simulink model "DSPequivalent_IM"  (R2018b)
settings: Solver=ode5  StartTime=0.0  StopTime=0.15  FixedStep=Tsim  RelTol=1e-3
values from neighbouring files (symbols this model uses):
  DEADTIME = 100    [init_DSPeq_FOC.m]    (also in init_DSPeq_IM.m)
  f_ref = 270    [init_DSPeq_FOC.m]    (also in init_DSPeq_IM.m = 50)
  Id_ref = 0    [init_DSPeq_FOC.m]    (also in init_DSPeq_IM.m = 1; step_prikaz.m = Idq2(:,2))
  Iq_ref = 2    [init_DSPeq_FOC.m]    (also in init_DSPeq_IM.m = 1; step_prikaz.m = Idq2(:,3))
  ISENSE_SCALE = 10    [init_DSPeq_FOC.m]    (also in init_DSPeq_IM.m)
  J = 15e-3    (= 0.015)    [init_DSPeq_IM.m]
  K1 = alpha*L/Ts    (= 68.108974359)    [init_DSPeq_FOC.m]    (also in init_DSPeq_IM.m = 301.121794872)
  K2 = exp(-Ts/taus)    [init_DSPeq_FOC.m]    (also in init_DSPeq_IM.m = exp(-Ts*Rs/Ls))
  Lge = (Ls*Lr-Lm^2)/Lr    (= 0.0459761697497)    [init_DSPeq_IM.m]
  Lm = 0.3482    [init_DSPeq_IM.m]
  Lr = Lm + Lgr    (= 0.3676)    [init_DSPeq_IM.m]
  Nos = 16    [init_DSPeq.m]    (also in init_DSPeq_FOC.m; init_DSPeq_IM.m)
  OVERSAMPLING = 1    [init_DSPeq.m]    (also in init_DSPeq_FOC.m; init_DSPeq_IM.m; raw_plot.m)
  p = 3    [init_DSPeq_FOC.m]    (also in init_DSPeq_IM.m = 1)
  PWM_TBPRD = 4992    [init_DSPeq.m]    (also in init_DSPeq_FOC.m; init_DSPeq_IM.m; paramSet.m)
  Rr = 11.202    [init_DSPeq_IM.m]
  Rs = 10    [init_DSPeq.m]    (also in init_DSPeq_IM.m = 13.12)
  Tadc = Tpwm/Nos    (= 6.24e-06)    [init_DSPeq.m]    (also in init_DSPeq_FOC.m; init_DSPeq_IM.m)
  Tpwm = 2*PWM_TBPRD/ftbclk    (= 9.984e-05)    [init_DSPeq.m]    (also in init_DSPeq_FOC.m; init_DSPeq_IM.m; paramSet.m)
  Ts = Tpwm/ur    (= 2.496e-05)    [init_DSPeq.m]    (also in init_DSPeq_FOC.m = 1.248e-05; init_DSPeq_IM.m = 4.992e-05; paramSet.m = 4.992e-05; step_prikaz.m = Ts/1000)
  Ttbclk = 1/ftbclk    (= 1e-08)    [init_DSPeq.m]    (also in init_DSPeq_FOC.m; init_DSPeq_IM.m; paramSet.m)
  UD_MAX = Udq_max    [init_DSPeq_IM.m]
  UD_MIN = -Udq_max    [init_DSPeq_IM.m]
  Udol = 0    [init_DSPeq_FOC.m]    (also in init_DSPeq_IM.m = UD_MAX/2)
  UQ_MAX = Udq_max    [init_DSPeq_IM.m]
  UQ_MIN = -Udq_max    [init_DSPeq_IM.m]
  Uqol = 0    [init_DSPeq_FOC.m]    (also in init_DSPeq_IM.m)
  ur = 4    [init_DSPeq.m]    (also in init_DSPeq_FOC.m = 8; init_DSPeq_IM.m = 2; paramSet.m = 2; raw_plot.m = 2)
libraries: simulink x7, simulink_extras x1
settings Model: Creator=ruzic  LastModifiedBy=ruzic
settings DebuggingCC: UnderSpecifiedDataTypeMsg=warning  UnderSpecifiedDimensionMsg=warning

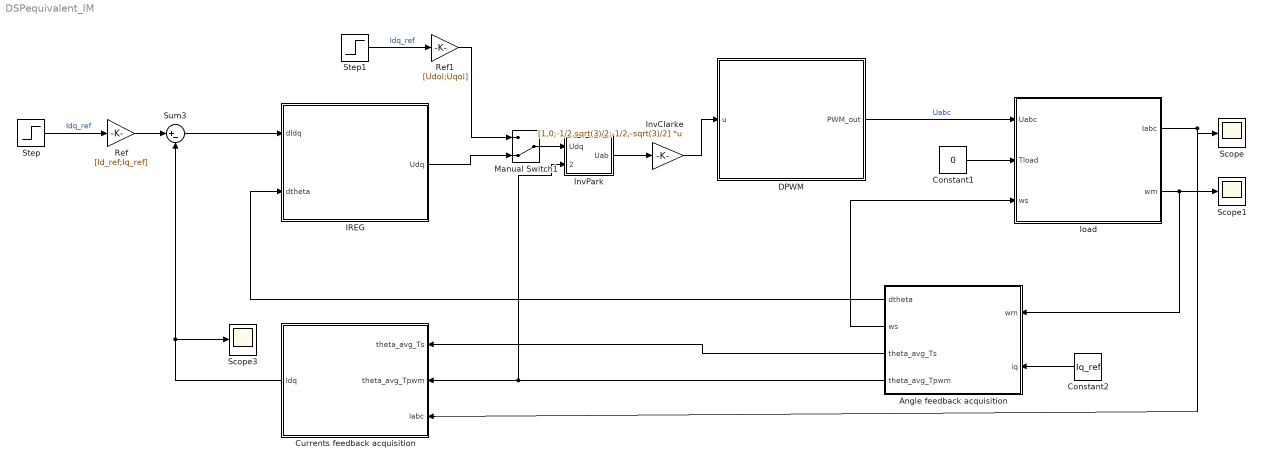
== system DSPequivalent_IM ==
  Angle feedback acquisition : Subsystem
  Constant1 : Constant  Value=0
  Constant2 : Constant  Value=Iq_ref
  Currents feedback acquisition : Subsystem
  DPWM : Subsystem
  IREG : Subsystem
  InvClarke : Gain  Gain=[1,0;-1/2,sqrt(3)/2;-1/2,-sqrt(3)/2]  Multiplication=Matrix(K*u)
  InvPark : Subsystem
  Manual Switch1 : ManualSwitch  CurrentSetting=0
  Ref : Gain  Gain=[Id_ref;Iq_ref]
  Ref1 : Gain  Gain=[Udol;Uqol]
  Scope : Scope
  Scope1 : Scope
  Scope3 : Scope
  Step : Step  Time=Tpwm/ur  SampleTime=Ts
  Step1 : Step  Time=Tpwm/ur  SampleTime=Ts
  Sum3 : Sum  Inputs=|+-
  load : Subsystem
  wires:
  Sum3/1 -> IREG/1(dIdq)
  Step/1 -> Ref/1  "Idq_ref"
  DPWM/1(PWM_out) -> load/1(Uabc)  "Uabc"
  load/1(Iabc) -> Scope/1, Currents feedback acquisition/3(Iabc)
  Ref1/1 -> Manual Switch1/1
  InvPark/1(Uab) -> InvClarke/1
  InvClarke/1 -> DPWM/1(u)
  Ref/1 -> Sum3/1
  Step1/1 -> Ref1/1  "Idq_ref"
  Currents feedback acquisition/1("Idq ") -> Scope3/1, Sum3/2
  IREG/1(Udq) -> Manual Switch1/2
  Manual Switch1/1 -> InvPark/1(Udq)
  Constant1/1 -> load/2(Tload)
  Angle feedback acquisition/4(theta_avg_Tpwm) -> Currents feedback acquisition/2(theta_avg_Tpwm), InvPark/2(theta)
  Angle feedback acquisition/1(dtheta) -> IREG/2(dtheta)
  Angle feedback acquisition/2(ws) -> load/3(ws)
  Angle feedback acquisition/3(theta_avg_Ts) -> Currents feedback acquisition/1(theta_avg_Ts)
  Constant2/1 -> Angle feedback acquisition/2(iq)
  load/2(wm) -> Angle feedback acquisition/1(wm), Scope1/1

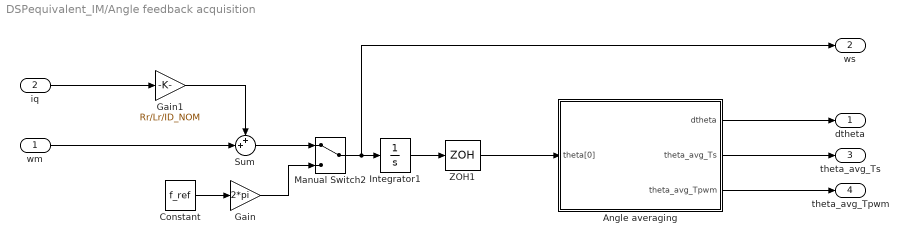
== system DSPequivalent_IM/Angle feedback acquisition ==
  wm : Inport
  iq : Inport  Port=2
  Angle averaging : Subsystem
  Constant : Constant  Value=f_ref
  Gain : Gain  Gain=2*pi
  Gain1 : Gain  Gain=Rr/Lr/ID_NOM
  Integrator1 : Integrator  WrapState=on  WrappedStateUpperValue=2*pi  WrappedStateLowerValue=0
  Manual Switch2 : ManualSwitch
  Sum : Sum  Inputs=++|
  ZOH1 : ZeroOrderHold  SampleTime=Ts
  dtheta : Outport
  ws : Outport  Port=2
  theta_avg_Ts : Outport  Port=3
  theta_avg_Tpwm : Outport  Port=4
  wires:
  ZOH1/1 -> Angle averaging/1(theta[0])
  Gain1/1 -> Sum/1
  iq/1 -> Gain1/1
  Sum/1 -> Manual Switch2/1
  Constant/1 -> Gain/1
  Manual Switch2/1 -> ws/1, Integrator1/1
  Gain/1 -> Manual Switch2/2
  Angle averaging/2(theta_avg_Ts) -> theta_avg_Ts/1
  Integrator1/1 -> ZOH1/1
  Angle averaging/3(theta_avg_Tpwm) -> theta_avg_Tpwm/1
  Angle averaging/1(dtheta) -> dtheta/1
  wm/1 -> Sum/2

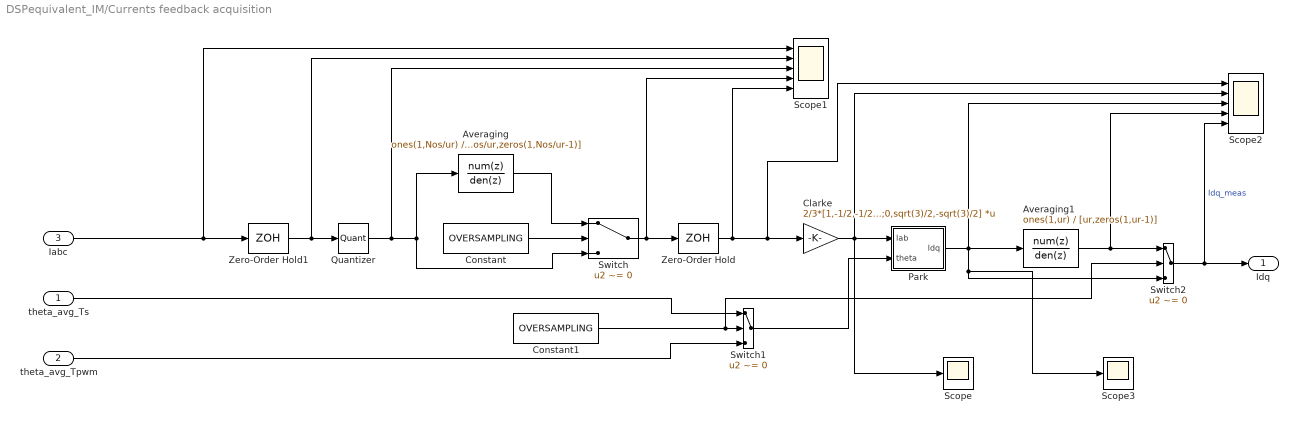
== system DSPequivalent_IM/Currents feedback acquisition ==
  theta_avg_Ts : Inport
  theta_avg_Tpwm : Inport  Port=2
  Iabc : Inport  Port=3
  Averaging : DiscreteTransferFcn  Numerator=ones(1,Nos/ur)  Denominator=[Nos/ur,zeros(1,Nos/ur-1)]
  Averaging1 : DiscreteTransferFcn  Numerator=ones(1,ur)  Denominator=[ur,zeros(1,ur-1)]
  Clarke : Gain  Gain=2/3*[1,-1/2,-1/2;0,sqrt(3)/2,-sqrt(3)/2]  Multiplication=Matrix(K*u)
  Constant : Constant  Value=OVERSAMPLING
  Constant1 : Constant  Value=OVERSAMPLING
  Park : Subsystem
  Quantizer : Quantizer  QuantizationInterval=3/(2^12-1)*ISENSE_SCALE
  Scope : Scope
  Scope1 : Scope  NumInputPorts=5
  Scope2 : Scope  NumInputPorts=5
  Scope3 : Scope
  Switch : Switch  Criteria=u2 ~= 0
  Switch1 : Switch  Criteria=u2 ~= 0
  Switch2 : Switch  Criteria=u2 ~= 0
  Zero-Order Hold : ZeroOrderHold  SampleTime=Ts
  Zero-Order Hold1 : ZeroOrderHold  SampleTime=Tadc
  "Idq " : Outport
  wires:
  Iabc/1 -> Zero-Order Hold1/1, Scope1/1
  Switch/1 -> Scope1/4, Zero-Order Hold/1
  Zero-Order Hold1/1 -> Quantizer/1, Scope1/2
  Quantizer/1 -> Switch/3, Averaging/1, Scope1/3
  Averaging/1 -> Switch/1
  Constant/1 -> Switch/2
  Constant1/1 -> Switch2/2, Switch1/2
  Switch2/1 -> Scope2/5, "Idq "/1  "Idq_meas"
  theta_avg_Tpwm/1 -> Switch1/3
  theta_avg_Ts/1 -> Switch1/1
  Averaging1/1 -> Scope2/4, Switch2/1
  Switch1/1 -> Park/2(theta)
  Clarke/1 -> Scope/1, Scope2/2, Park/1(Iab)
  Park/1(Idq) -> Scope2/3, Averaging1/1, Scope3/1, Switch2/3
  Zero-Order Hold/1 -> Scope2/1, Clarke/1, Scope1/5

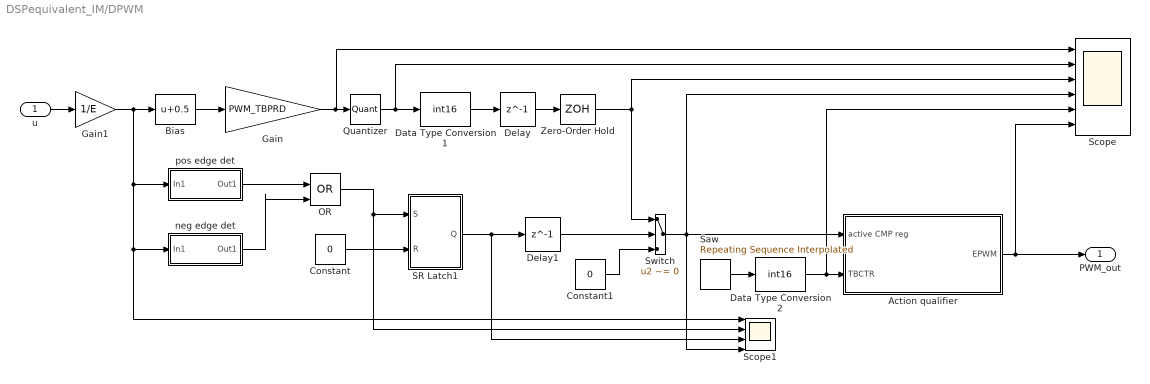
== system DSPequivalent_IM/DPWM ==
  u : Inport
  Action qualifier : Subsystem
  Bias : Bias  Bias=0.5
  Constant : Constant  Value=0
  Constant1 : Constant  Value=0
  Data Type Conversion1 : DataTypeConversion  OutDataTypeStr=int16  ConvertRealWorld=Stored Integer (SI)  RndMeth=Round
  Data Type Conversion2 : DataTypeConversion  OutDataTypeStr=int16  ConvertRealWorld=Stored Integer (SI)  RndMeth=Round
  Delay : Delay  DelayLength=1  SampleTime=Ts
  Delay1 : Delay  DelayLength=1  SampleTime=Ts
  Gain : Gain  Gain=PWM_TBPRD
  Gain1 : Gain  Gain=1/E
  OR : Logic  Operator=OR  IconShape=distinctive  AllPortsSameDT=off  OutDataTypeStr=boolean
  Quantizer : Quantizer  QuantizationInterval=1
  SR Latch1 : Subsystem
  Saw : simulink/Sources/Repeating Sequence Interpolated  OutValues=[0 PWM_TBPRD 1].'  TimeValues=[0 Tpwm/2 (Tpwm-Ttbclk)].'  LookUpMeth=Interpolation-Use End Values  tsamp=Ttbclk  OutMin=[]  OutMax=[]  OutDataTypeStr=double  OutputDataTypeScalingMode=double  OutDataType=fixdt(0,8)  OutScaling=2^-10
  Scope : Scope  NumInputPorts=6
  Scope1 : Scope  NumInputPorts=4
  Switch : Switch  Criteria=u2 ~= 0
  Zero-Order Hold : ZeroOrderHold  SampleTime=-1
  neg edge det : Subsystem
  pos edge det : Subsystem
  PWM_out : Outport
  wires:
  u/1 -> Gain1/1
  Quantizer/1 -> Data Type Conversion1/1, Scope/2
  Saw/1 -> Data Type Conversion2/1
  Switch/1 -> Scope/4, Action qualifier/1(active CMP reg), Scope1/4
  Action qualifier/1(EPWM) -> Scope/6, PWM_out/1
  Data Type Conversion1/1 -> Delay/1
  Data Type Conversion2/1 -> Scope/5, Action qualifier/2(TBCTR)
  Gain1/1 -> Scope1/1, neg edge det/1(In1), pos edge det/1(In1), Bias/1
  Gain/1 -> Scope/1, Quantizer/1
  Constant/1 -> SR Latch1/2(R)
  neg edge det/1(Out1) -> OR/2
  pos edge det/1(Out1) -> OR/1
  OR/1 -> Scope1/2, SR Latch1/1(S)
  SR Latch1/1(Q) -> Scope1/3, Delay1/1
  Constant1/1 -> Switch/3
  Bias/1 -> Gain/1
  Delay/1 -> Zero-Order Hold/1
  Zero-Order Hold/1 -> Scope/3, Switch/1
  Delay1/1 -> Switch/2

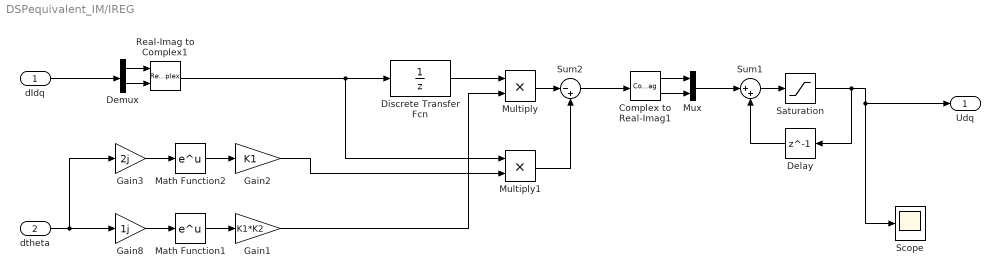
== system DSPequivalent_IM/IREG ==
  dIdq : Inport
  dtheta : Inport  Port=2
  Complex to Real-Imag1 : ComplexToRealImag
  Delay : Delay  DelayLength=1
  Demux : Demux  Outputs=2
  Discrete Transfer Fcn : DiscreteTransferFcn  Denominator=[1 0]
  Gain1 : Gain  Gain=K1*K2
  Gain2 : Gain  Gain=K1
  Gain3 : Gain  Gain=2j
  Gain8 : Gain  Gain=1j
  Math Function1 : Math  OutputSignalType=complex  SaturateOnIntegerOverflow=on
  Math Function2 : Math  OutputSignalType=complex  SaturateOnIntegerOverflow=on
  Multiply : Product
  Multiply1 : Product
  Mux : Mux  Inputs=2
  Real-Imag to Complex1 : RealImagToComplex
  Saturation : Saturate  UpperLimit=[UD_MAX; UQ_MAX]  LowerLimit=[UD_MIN; UQ_MIN]
  Scope : Scope
  Sum1 : Sum  Inputs=|++
  Sum2 : Sum  Inputs=|-+
  Udq : Outport
  wires:
  Saturation/1 -> Udq/1, Scope/1, Delay/1
  Sum1/1 -> Saturation/1
  Delay/1 -> Sum1/2
  Demux/2 -> Real-Imag to Complex1/2
  Math Function1/1 -> Gain1/1
  Mux/1 -> Sum1/1
  Gain3/1 -> Math Function2/1
  Gain8/1 -> Math Function1/1
  dtheta/1 -> Gain3/1, Gain8/1
  Demux/1 -> Real-Imag to Complex1/1
  Real-Imag to Complex1/1 -> Discrete Transfer Fcn/1, Multiply1/1
  dIdq/1 -> Demux/1
  Math Function2/1 -> Gain2/1
  Gain1/1 -> Multiply/2
  Sum2/1 -> Complex to Real-Imag1/1
  Complex to Real-Imag1/2 -> Mux/2
  Complex to Real-Imag1/1 -> Mux/1
  Multiply/1 -> Sum2/1
  Gain2/1 -> Multiply1/2
  Multiply1/1 -> Sum2/2
  Discrete Transfer Fcn/1 -> Multiply/1

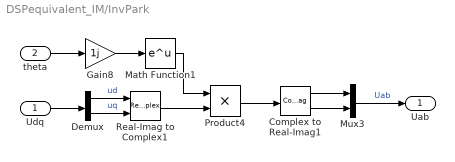
== system DSPequivalent_IM/InvPark ==
  Udq : Inport
  theta : Inport  Port=2
  Complex to Real-Imag1 : ComplexToRealImag
  Demux : Demux  Outputs=2
  Gain8 : Gain  Gain=1j
  Math Function1 : Math  OutputSignalType=complex  SaturateOnIntegerOverflow=on
  Mux3 : Mux  Inputs=2
  Product4 : Product
  Real-Imag to Complex1 : RealImagToComplex
  Uab : Outport
  wires:
  Real-Imag to Complex1/1 -> Product4/2
  Math Function1/1 -> Product4/1
  Complex to Real-Imag1/1 -> Mux3/1
  Gain8/1 -> Math Function1/1
  Demux/1 -> Real-Imag to Complex1/1  "ud"
  Mux3/1 -> Uab/1  "Uab"
  Product4/1 -> Complex to Real-Imag1/1
  Complex to Real-Imag1/2 -> Mux3/2
  Demux/2 -> Real-Imag to Complex1/2  "uq"
  theta/1 -> Gain8/1
  Udq/1 -> Demux/1

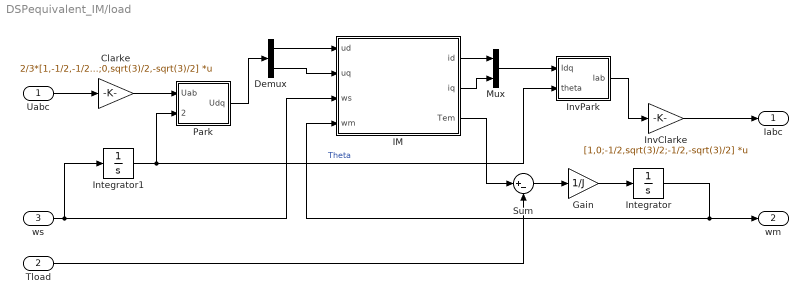
== system DSPequivalent_IM/load ==
  Uabc : Inport
  Tload : Inport  Port=2
  ws : Inport  Port=3
  Clarke : Gain  Gain=2/3*[1,-1/2,-1/2;0,sqrt(3)/2,-sqrt(3)/2]  Multiplication=Matrix(K*u)
  Demux : Demux  Outputs=2
  Gain : Gain  Gain=1/J
  IM : Subsystem
  Integrator : Integrator
  Integrator1 : Integrator  WrapState=on  WrappedStateUpperValue=2*pi  WrappedStateLowerValue=0
  InvClarke : Gain  Gain=[1,0;-1/2,sqrt(3)/2;-1/2,-sqrt(3)/2]  Multiplication=Matrix(K*u)
  InvPark : Subsystem
  Mux : Mux  Inputs=2
  Park : Subsystem
  Sum : Sum  Inputs=|+-
  Iabc : Outport
  wm : Outport  Port=2
  wires:
  Uabc/1 -> Clarke/1
  Clarke/1 -> Park/1(Uab)
  Park/1(Udq) -> Demux/1
  Demux/1 -> IM/1(ud)
  Demux/2 -> IM/2(uq)
  InvPark/1(Iab) -> InvClarke/1
  Mux/1 -> InvPark/1(Idq)
  InvClarke/1 -> Iabc/1
  IM/1(id) -> Mux/1
  IM/2(iq) -> Mux/2
  IM/3(Tem) -> Sum/1
  Sum/1 -> Gain/1
  Gain/1 -> Integrator/1
  Tload/1 -> Sum/2
  Integrator/1 -> IM/4(wm), wm/1
  ws/1 -> IM/3(ws), Integrator1/1
  Integrator1/1 -> Park/2(theta), InvPark/2(theta)  "Theta"

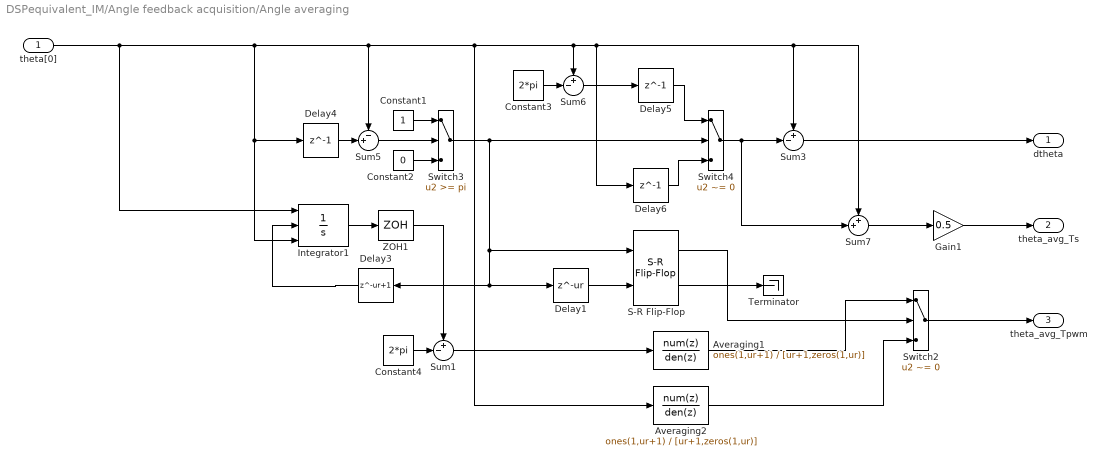
== system DSPequivalent_IM/Angle feedback acquisition/Angle averaging ==
  theta[0] : Inport
  Averaging1 : DiscreteTransferFcn  Numerator=ones(1,ur+1)  Denominator=[ur+1,zeros(1,ur)]  SampleTime=Ts
  Averaging2 : DiscreteTransferFcn  Numerator=ones(1,ur+1)  Denominator=[ur+1,zeros(1,ur)]  SampleTime=Ts
  Constant1 : Constant
  Constant2 : Constant  Value=0
  Constant3 : Constant  Value=2*pi
  Constant4 : Constant  Value=2*pi
  Delay1 : Delay  DelayLength=ur  SampleTime=Ts
  Delay3 : Delay  DelayLength=ur+1  SampleTime=Ts
  Delay4 : Delay  DelayLength=1
  Delay5 : Delay  DelayLength=1  SampleTime=Ts
  Delay6 : Delay  DelayLength=1  SampleTime=Ts
  Gain1 : Gain  Gain=0.5
  Integrator1 : Integrator  ExternalReset=rising  InitialConditionSource=external  InitialCondition=5
  S-R Flip-Flop : simulink_extras/Flip Flops/S-R Flip-Flop  initial_condition=0
  Sum1 : Sum  Inputs=+-|
  Sum3 : Sum  Inputs=+-|
  Sum5 : Sum  Inputs=-+|
  Sum6 : Sum  Inputs=+-|
  Sum7 : Sum  Inputs=++|
  Switch2 : Switch  Criteria=u2 ~= 0
  Switch3 : Switch  Threshold=pi  OutDataTypeStr=boolean
  Switch4 : Switch  Criteria=u2 ~= 0
  Terminator : Terminator
  ZOH1 : ZeroOrderHold  SampleTime=Ts
  dtheta : Outport
  theta_avg_Ts : Outport  Port=2
  theta_avg_Tpwm : Outport  Port=3
  wires:
  Sum3/1 -> dtheta/1
  Delay4/1 -> Sum5/2
  Sum5/1 -> Switch3/2
  Constant1/1 -> Switch3/1
  Constant2/1 -> Switch3/3
  Constant3/1 -> Sum6/2
  Switch3/1 -> Delay3/1, Delay1/1, S-R Flip-Flop/1, Switch4/2
  Delay5/1 -> Switch4/1
  Switch4/1 -> Sum7/2, Sum3/2
  Delay6/1 -> Switch4/3
  Sum7/1 -> Gain1/1
  Sum6/1 -> Delay5/1
  Gain1/1 -> theta_avg_Ts/1
  S-R Flip-Flop/2 -> Terminator/1
  Delay1/1 -> S-R Flip-Flop/2
  S-R Flip-Flop/1 -> Switch2/2
  Integrator1/1 -> ZOH1/1
  theta[0]/1 -> Averaging2/1, Delay6/1, Sum7/1, Sum3/1, Sum6/1, Sum5/1, Integrator1/3, Delay4/1, Integrator1/1
  Delay3/1 -> Integrator1/2
  Switch2/1 -> theta_avg_Tpwm/1
  Averaging1/1 -> Switch2/1
  Averaging2/1 -> Switch2/3
  Constant4/1 -> Sum1/2
  ZOH1/1 -> Sum1/1
  Sum1/1 -> Averaging1/1

== system DSPequivalent_IM/Currents feedback acquisition/Park ==
  Iab : Inport
  theta : Inport  Port=2
  Complex to Real-Imag1 : ComplexToRealImag
  Demux : Demux  Outputs=2
  Gain8 : Gain  Gain=-1j
  Math Function1 : Math  OutputSignalType=complex  SaturateOnIntegerOverflow=on
  Mux3 : Mux  Inputs=2
  Product4 : Product
  Real-Imag to Complex1 : RealImagToComplex
  Idq : Outport
  wires:
  Real-Imag to Complex1/1 -> Product4/2
  Math Function1/1 -> Product4/1
  Complex to Real-Imag1/1 -> Mux3/1
  Gain8/1 -> Math Function1/1
  theta/1 -> Gain8/1
  Demux/1 -> Real-Imag to Complex1/1  "ialfa"
  Mux3/1 -> Idq/1  "Idq"
  Product4/1 -> Complex to Real-Imag1/1
  Complex to Real-Imag1/2 -> Mux3/2
  Demux/2 -> Real-Imag to Complex1/2  "ibeta"
  Iab/1 -> Demux/1

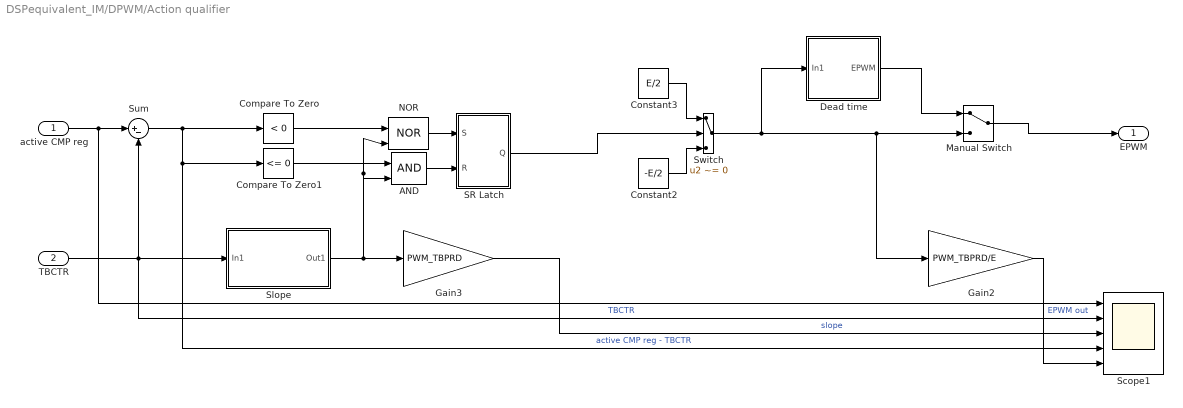
== system DSPequivalent_IM/DPWM/Action qualifier ==
  active CMP reg : Inport
  TBCTR : Inport  Port=2
  AND : Logic  IconShape=distinctive  AllPortsSameDT=off  OutDataTypeStr=boolean
  Compare To Zero : simulink/Logic and Bit Operations/Compare To Zero  relop=<  OutDataTypeStr=boolean
  Compare To Zero1 : simulink/Logic and Bit Operations/Compare To Zero  relop=<=  OutDataTypeStr=boolean
  Constant2 : Constant  Value=-E/2
  Constant3 : Constant  Value=E/2
  Dead time : Subsystem
  Gain2 : Gain  Gain=PWM_TBPRD/E
  Gain3 : Gain  Gain=PWM_TBPRD
  Manual Switch : ManualSwitch
  NOR : Logic  Operator=NOR  IconShape=distinctive  AllPortsSameDT=off  OutDataTypeStr=boolean
  SR Latch : Subsystem
  Scope1 : Scope  NumInputPorts=5
  Slope : Subsystem
  Sum : Sum  Inputs=|+-
  Switch : Switch  Criteria=u2 ~= 0
  EPWM : Outport
  wires:
  Gain3/1 -> Scope1/3  "slope"
  active CMP reg/1 -> Scope1/1, Sum/1
  Gain2/1 -> Scope1/5  "EPWM out"
  Sum/1 -> Scope1/4, Compare To Zero1/1, Compare To Zero/1  "active CMP reg - TBCTR"
  TBCTR/1 -> Scope1/2, Slope/1(In1), Sum/2  "TBCTR"
  AND/1 -> SR Latch/2(R)
  Compare To Zero/1 -> NOR/1
  NOR/1 -> SR Latch/1(S)
  Compare To Zero1/1 -> AND/1
  Slope/1(Out1) -> Gain3/1, AND/2, NOR/2
  SR Latch/1(Q) -> Switch/2
  Constant2/1 -> Switch/3
  Constant3/1 -> Switch/1
  Manual Switch/1 -> EPWM/1
  Dead time/1(EPWM) -> Manual Switch/1
  Switch/1 -> Manual Switch/2, Gain2/1, Dead time/1(In1)

== system DSPequivalent_IM/DPWM/SR Latch1 ==
  S : Inport
  R : Inport  Port=2
  AND1 : Logic  IconShape=distinctive  AllPortsSameDT=off  OutDataTypeStr=boolean
  Memory : Memory
  NOT : Logic  Operator=NOT  IconShape=distinctive  AllPortsSameDT=off  OutDataTypeStr=boolean
  OR : Logic  Operator=OR  IconShape=distinctive  AllPortsSameDT=off  OutDataTypeStr=boolean
  Q : Outport
  wires:
  AND1/1 -> Q/1, Memory/1
  R/1 -> NOT/1
  S/1 -> OR/2
  OR/1 -> AND1/1
  NOT/1 -> AND1/2
  Memory/1 -> OR/1

== system DSPequivalent_IM/DPWM/neg edge det ==
  In1 : Inport
  AND : Logic  IconShape=distinctive  AllPortsSameDT=off  OutDataTypeStr=boolean
  Memory : Memory
  NOT : Logic  Operator=NOT  IconShape=distinctive  AllPortsSameDT=off  OutDataTypeStr=boolean
  Out1 : Outport
  wires:
  Memory/1 -> AND/1
  In1/1 -> NOT/1, Memory/1
  AND/1 -> Out1/1
  NOT/1 -> AND/2

== system DSPequivalent_IM/DPWM/pos edge det ==
  In1 : Inport
  AND : Logic  IconShape=distinctive  AllPortsSameDT=off  OutDataTypeStr=boolean
  Memory : Memory
  NOT : Logic  Operator=NOT  IconShape=distinctive  AllPortsSameDT=off  OutDataTypeStr=boolean
  Out1 : Outport
  wires:
  NOT/1 -> AND/1
  Memory/1 -> NOT/1
  In1/1 -> AND/2, Memory/1
  AND/1 -> Out1/1

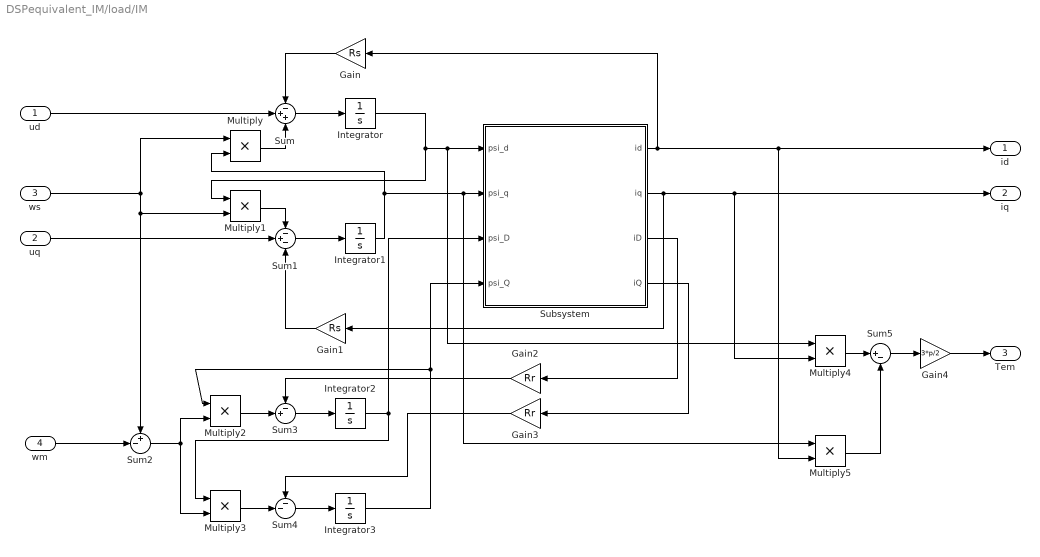
== system DSPequivalent_IM/load/IM ==
  ud : Inport
  uq : Inport  Port=2
  ws : Inport  Port=3
  wm : Inport  Port=4
  Gain : Gain  Gain=Rs
  Gain1 : Gain  Gain=Rs
  Gain2 : Gain  Gain=Rr
  Gain3 : Gain  Gain=Rr
  Gain4 : Gain  Gain=3*p/2
  Integrator{,1..3} (4 alike) : Integrator
  Multiply{,1..5} (6 alike) : Product
  Subsystem : Subsystem
  Sum : Sum  Inputs=-++
  Sum1 : Sum  Inputs=-+-
  Sum2 : Sum  Inputs=+-|
  Sum3 : Sum  Inputs=-+|
  Sum4 : Sum  Inputs=--|
  Sum5 : Sum  Inputs=|+-
  id : Outport
  iq : Outport  Port=2
  Tem : Outport  Port=3
  wires:
  Sum2/1 -> Multiply3/2, Multiply2/2
  Integrator/1 -> Multiply4/1, Subsystem/1(psi_d), Multiply1/1
  Integrator2/1 -> Subsystem/3(psi_D), Multiply3/1
  Integrator3/1 -> Multiply2/1, Subsystem/4(psi_Q)
  Subsystem/3(iD) -> Gain2/1
  ud/1 -> Sum/2
  ws/1 -> Multiply1/2, Sum2/1, Multiply/1
  Subsystem/4(iQ) -> Gain3/1
  Multiply3/1 -> Sum4/2
  Gain3/1 -> Sum4/1
  Multiply/1 -> Sum/3
  Gain2/1 -> Sum3/1
  Sum4/1 -> Integrator3/1
  Sum1/1 -> Integrator1/1
  Integrator1/1 -> Multiply5/1, Subsystem/2(psi_q), Multiply/2
  Sum3/1 -> Integrator2/1
  Multiply2/1 -> Sum3/2
  Subsystem/1(id) -> id/1, Multiply5/2, Gain/1
  Subsystem/2(iq) -> iq/1, Multiply4/2, Gain1/1
  wm/1 -> Sum2/2
  Sum/1 -> Integrator/1
  Gain1/1 -> Sum1/3
  Gain/1 -> Sum/1
  uq/1 -> Sum1/2
  Multiply1/1 -> Sum1/1
  Sum5/1 -> Gain4/1
  Multiply4/1 -> Sum5/1
  Gain4/1 -> Tem/1
  Multiply5/1 -> Sum5/2

== system DSPequivalent_IM/load/InvPark ==
  Idq : Inport
  theta : Inport  Port=2
  Complex to Real-Imag1 : ComplexToRealImag
  Demux : Demux  Outputs=2
  Gain8 : Gain  Gain=1j
  Math Function1 : Math  OutputSignalType=complex  SaturateOnIntegerOverflow=on
  Mux3 : Mux  Inputs=2
  Product4 : Product
  Real-Imag to Complex1 : RealImagToComplex
  Iab : Outport
  wires:
  Real-Imag to Complex1/1 -> Product4/2
  Math Function1/1 -> Product4/1
  Complex to Real-Imag1/1 -> Mux3/1
  Gain8/1 -> Math Function1/1
  Demux/1 -> Real-Imag to Complex1/1  "ud"
  Mux3/1 -> Iab/1  "Uab"
  Product4/1 -> Complex to Real-Imag1/1
  Complex to Real-Imag1/2 -> Mux3/2
  Demux/2 -> Real-Imag to Complex1/2  "uq"
  theta/1 -> Gain8/1
  Idq/1 -> Demux/1

== system DSPequivalent_IM/load/Park ==
  Uab : Inport
  theta : Inport  Port=2
  Complex to Real-Imag1 : ComplexToRealImag
  Demux : Demux  Outputs=2
  Gain8 : Gain  Gain=-1j
  Math Function1 : Math  OutputSignalType=complex  SaturateOnIntegerOverflow=on
  Mux3 : Mux  Inputs=2
  Product4 : Product
  Real-Imag to Complex1 : RealImagToComplex
  Udq : Outport
  wires:
  Real-Imag to Complex1/1 -> Product4/2
  Math Function1/1 -> Product4/1
  Complex to Real-Imag1/1 -> Mux3/1
  Gain8/1 -> Math Function1/1
  theta/1 -> Gain8/1
  Demux/1 -> Real-Imag to Complex1/1  "ialfa"
  Mux3/1 -> Udq/1  "Udq"
  Product4/1 -> Complex to Real-Imag1/1
  Complex to Real-Imag1/2 -> Mux3/2
  Demux/2 -> Real-Imag to Complex1/2  "ibeta"
  Uab/1 -> Demux/1

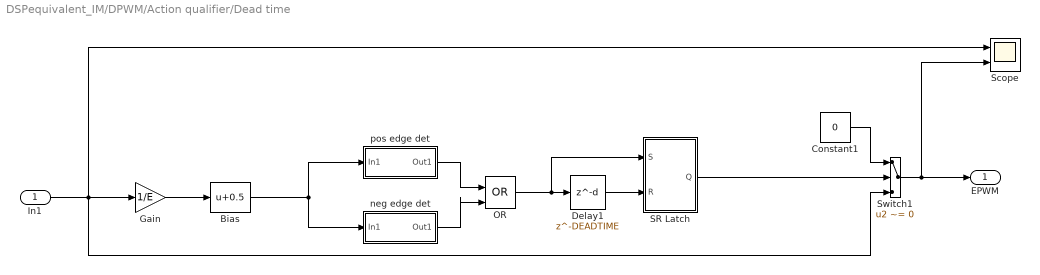
== system DSPequivalent_IM/DPWM/Action qualifier/Dead time ==
  In1 : Inport
  Bias : Bias  Bias=0.5
  Constant1 : Constant  Value=0
  Delay1 : Delay  DelayLength=DEADTIME  SampleTime=Ttbclk
  Gain : Gain  Gain=1/E
  OR : Logic  Operator=OR  IconShape=distinctive  AllPortsSameDT=off  OutDataTypeStr=boolean
  SR Latch : Subsystem
  Scope : Scope  NumInputPorts=2
  Switch1 : Switch  Criteria=u2 ~= 0
  neg edge det : Subsystem
  pos edge det : Subsystem
  EPWM : Outport
  wires:
  neg edge det/1(Out1) -> OR/2
  pos edge det/1(Out1) -> OR/1
  Delay1/1 -> SR Latch/2(R)
  OR/1 -> SR Latch/1(S), Delay1/1
  SR Latch/1(Q) -> Switch1/2
  Switch1/1 -> Scope/2, EPWM/1
  In1/1 -> Switch1/3, Scope/1, Gain/1
  Gain/1 -> Bias/1
  Bias/1 -> neg edge det/1(In1), pos edge det/1(In1)
  Constant1/1 -> Switch1/1

== system DSPequivalent_IM/DPWM/Action qualifier/SR Latch ==
  S : Inport
  R : Inport  Port=2
  AND1 : Logic  IconShape=distinctive  AllPortsSameDT=off  OutDataTypeStr=boolean
  Memory : Memory
  NOT : Logic  Operator=NOT  IconShape=distinctive  AllPortsSameDT=off  OutDataTypeStr=boolean
  OR : Logic  Operator=OR  IconShape=distinctive  AllPortsSameDT=off  OutDataTypeStr=boolean
  Q : Outport
  wires:
  AND1/1 -> Q/1, Memory/1
  R/1 -> NOT/1
  S/1 -> OR/2
  OR/1 -> AND1/1
  NOT/1 -> AND1/2
  Memory/1 -> OR/1

== system DSPequivalent_IM/DPWM/Action qualifier/Slope ==
  In1 : Inport
  AND : Logic  IconShape=distinctive  AllPortsSameDT=off  OutDataTypeStr=boolean
  Compare To Constant : simulink/Logic and Bit Operations/Compare To Constant  relop===  const=PWM_TBPRD  OutDataTypeStr=boolean
  Compare To Zero : simulink/Logic and Bit Operations/Compare To Zero  relop=~=  OutDataTypeStr=boolean
  Compare To Zero1 : simulink/Logic and Bit Operations/Compare To Zero  relop=<  OutDataTypeStr=boolean
  Difference : simulink/Discrete/Difference  ICPrevInput=0  OutMin=[]  OutMax=[]  OutDataTypeStr=int16  OutputDataTypeScalingMode=int16  OutDataType=fixdt(1, 16)  OutScaling=2^-10  DoSatur=off
  NOT : Logic  Operator=NOT  IconShape=distinctive  AllPortsSameDT=off  OutDataTypeStr=boolean
  OR : Logic  Operator=OR  IconShape=distinctive  AllPortsSameDT=off  OutDataTypeStr=boolean
  Out1 : Outport
  wires:
  In1/1 -> Difference/1, Compare To Constant/1, Compare To Zero/1
  AND/1 -> OR/1
  Compare To Zero1/1 -> AND/1
  Compare To Constant/1 -> OR/2
  Difference/1 -> Compare To Zero1/1
  OR/1 -> NOT/1
  Compare To Zero/1 -> AND/2
  NOT/1 -> Out1/1

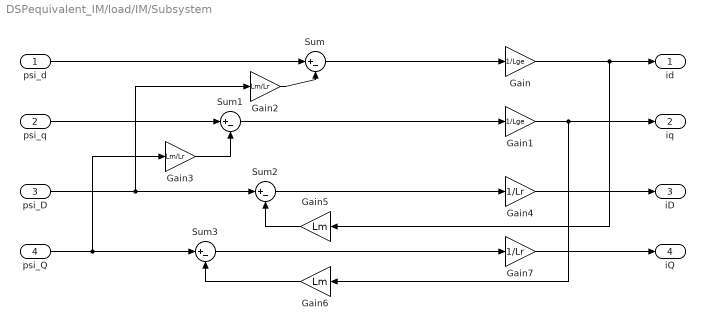
== system DSPequivalent_IM/load/IM/Subsystem ==
  psi_d : Inport
  psi_q : Inport  Port=2
  psi_D : Inport  Port=3
  psi_Q : Inport  Port=4
  Gain : Gain  Gain=1/Lge
  Gain1 : Gain  Gain=1/Lge
  Gain2 : Gain  Gain=Lm/Lr
  Gain3 : Gain  Gain=Lm/Lr
  Gain4 : Gain  Gain=1/Lr
  Gain5 : Gain  Gain=Lm
  Gain6 : Gain  Gain=Lm
  Gain7 : Gain  Gain=1/Lr
  Sum{,1..3} (4 alike) : Sum  Inputs=|+-
  id : Outport
  iq : Outport  Port=2
  iD : Outport  Port=3
  iQ : Outport  Port=4
  wires:
  psi_d/1 -> Sum/1
  Gain1/1 -> Gain6/1, iq/1
  Gain2/1 -> Sum/2
  Sum/1 -> Gain/1
  psi_Q/1 -> Sum3/1, Gain3/1
  psi_q/1 -> Sum1/1
  Gain3/1 -> Sum1/2
  Sum1/1 -> Gain1/1
  psi_D/1 -> Sum2/1, Gain2/1
  Gain4/1 -> iD/1
  Sum2/1 -> Gain4/1
  Gain/1 -> Gain5/1, id/1
  Gain5/1 -> Sum2/2
  Gain6/1 -> Sum3/2
  Sum3/1 -> Gain7/1
  Gain7/1 -> iQ/1

== system DSPequivalent_IM/DPWM/Action qualifier/Dead time/SR Latch ==
  S : Inport
  R : Inport  Port=2
  AND1 : Logic  IconShape=distinctive  AllPortsSameDT=off  OutDataTypeStr=boolean
  Memory : Memory
  NOT : Logic  Operator=NOT  IconShape=distinctive  AllPortsSameDT=off  OutDataTypeStr=boolean
  OR : Logic  Operator=OR  IconShape=distinctive  AllPortsSameDT=off  OutDataTypeStr=boolean
  Q : Outport
  wires:
  AND1/1 -> Q/1, Memory/1
  R/1 -> NOT/1
  S/1 -> OR/2
  OR/1 -> AND1/1
  NOT/1 -> AND1/2
  Memory/1 -> OR/1

== system DSPequivalent_IM/DPWM/Action qualifier/Dead time/neg edge det ==
  In1 : Inport
  AND : Logic  IconShape=distinctive  AllPortsSameDT=off  OutDataTypeStr=boolean
  Memory : Memory
  NOT : Logic  Operator=NOT  IconShape=distinctive  AllPortsSameDT=off  OutDataTypeStr=boolean
  Out1 : Outport
  wires:
  Memory/1 -> AND/1
  In1/1 -> NOT/1, Memory/1
  AND/1 -> Out1/1
  NOT/1 -> AND/2

== system DSPequivalent_IM/DPWM/Action qualifier/Dead time/pos edge det ==
  In1 : Inport
  AND : Logic  IconShape=distinctive  AllPortsSameDT=off  OutDataTypeStr=boolean
  Memory : Memory
  NOT : Logic  Operator=NOT  IconShape=distinctive  AllPortsSameDT=off  OutDataTypeStr=boolean
  Out1 : Outport
  wires:
  NOT/1 -> AND/1
  Memory/1 -> NOT/1
  In1/1 -> AND/2, Memory/1
  AND/1 -> Out1/1
